simulink model "DKSTDD_DK_TuanTu_SG_Q_P_Y"  (R2019a)
settings: Solver=VariableStepAuto  StartTime=0.0  StopTime=10  RelTol=1e-3
libraries: powerlib x8
settings Model: Creator=Admin  LastModifiedBy=Admin
settings SolverCC: ZeroCrossAlgorithm=Adaptive
settings DebuggingCC: IgnoredZcDiagnostic=none

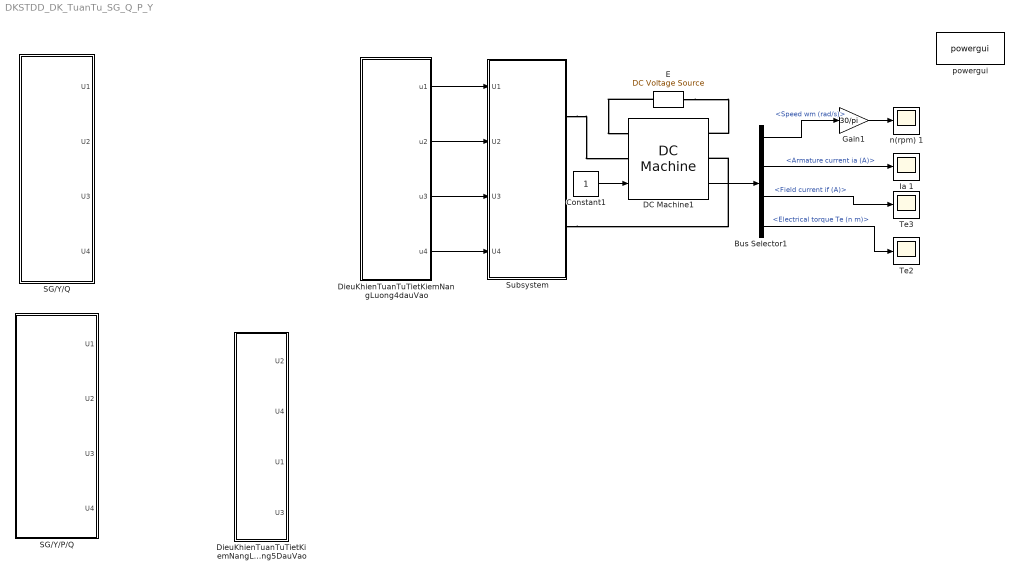
== system DKSTDD_DK_TuanTu_SG_Q_P_Y ==
  Bus Selector1 : BusSelector  OutputSignals=Speed wm (rad/s),Armature current ia (A),Field current if (A),Electrical torque Te (n m)
  Constant1 : Constant
  DC Machine1 : powerlib/Machines/DC Machine  PresetModel=01: 5HP 240V 1750RPM Field:300V  MechanicalLoad=Torque TL  FieldType=Wound  ShowDetailedParameters=on  MeasurementBus=off  RLa=[2.581 0.028]  RLf=[281.3 156]  Laf=0.9483  MachineConstant=Torque constant (N.m/A)  Ke=1.8  Kt=1.8  J=0.02215  Bm=0.002953  Tf=0.5161  w0=1  Ifinit=1  TsPowergui=0  TsBlock=-1
  "DieuKhienTuanTuTietKiemNangLuong4dauVao " : Subsystem
  "DieuKhienTuanTuTietKiemNangLuong5DauVao " : Subsystem
  E : powerlib/Electrical Sources/DC Voltage Source  Amplitude=300  Measurements=None
  Gain1 : Gain  Gain=30/pi
  Ia 1 : Scope
  SG/Y/P/Q : Subsystem
  SG/Y/Q : Subsystem
  Subsystem : Subsystem
  Te2 : Scope
  Te3 : Scope
  n(rpm) 1 : Scope
  powergui : powerlib/powergui  Priority=1  SimulationMode=Continuous  SampleTime=50e-6  frequency=60  Iterations=50  frequencyindice=0  Pbase=100e6  ErrMax=1e-4  UnitsV=kV  UnitsW=MW  buscounter=0  FunctionMessages=off  echomessages=off  EnableUseOfTLC=off  CurrentSourceSwitches=off  DisableSnubberDevices=off  DisableRonSwitches=off  DisableVfSwitches=off  DisplayEquations=off  AutomaticDiscreteSolvers=off  SolverType=Tustin/Backward Euler (TBE)  Interpol=off  ExternalGateDelay=off  methode=off  Ts=100  x0status=blocks  SPID=on  SwTol=0  HookPort=off  NonlinearTolerance=0  nMaxIteration=15  ContinueOnMaxIteration=off  RestoreLinks=warning  ResistiveCurrentMeasurement=off  Frange=[0:2:500]  Ylog=off  Xlog=on  ShowGrid=off  save=off  variable=ZData  structure=0  ZoomFFT=off  StartTime=0.0  cycles=1  DisplayStyle=1  fundamental=60  FreqAxis=off  MaxFrequency=1000  frequencyindicesteady=1  RmsSteady=1  display=off
      settings: SourceProductName=Simscape Electrical
  wires:
  Bus Selector1/4 -> Te2/1  "<Electrical torque Te (n m)>"
  Gain1/1 -> n(rpm) 1/1
  DC Machine1/1 -> Bus Selector1/1
  Bus Selector1/3 -> Te3/1  "<Field current if (A)>"
  Bus Selector1/1 -> Gain1/1  "<Speed wm (rad/s)>"
  Constant1/1 -> DC Machine1/1
  Bus Selector1/2 -> Ia 1/1  "<Armature current ia (A)>"
  "DieuKhienTuanTuTietKiemNangLuong4dauVao "/1(u1) -> Subsystem/1(U1)
  "DieuKhienTuanTuTietKiemNangLuong4dauVao "/2("u2 ") -> Subsystem/2(U2)
  "DieuKhienTuanTuTietKiemNangLuong4dauVao "/3(u3) -> Subsystem/3(U3)
  "DieuKhienTuanTuTietKiemNangLuong4dauVao "/4(u4) -> Subsystem/4(U4)
  connections:
  E/RConn1 -- DC Machine1/LConn2
  Subsystem/RConn2 -- DC Machine1/RConn1
  Subsystem/RConn1 -- DC Machine1/LConn1
  E/LConn1 -- DC Machine1/RConn2

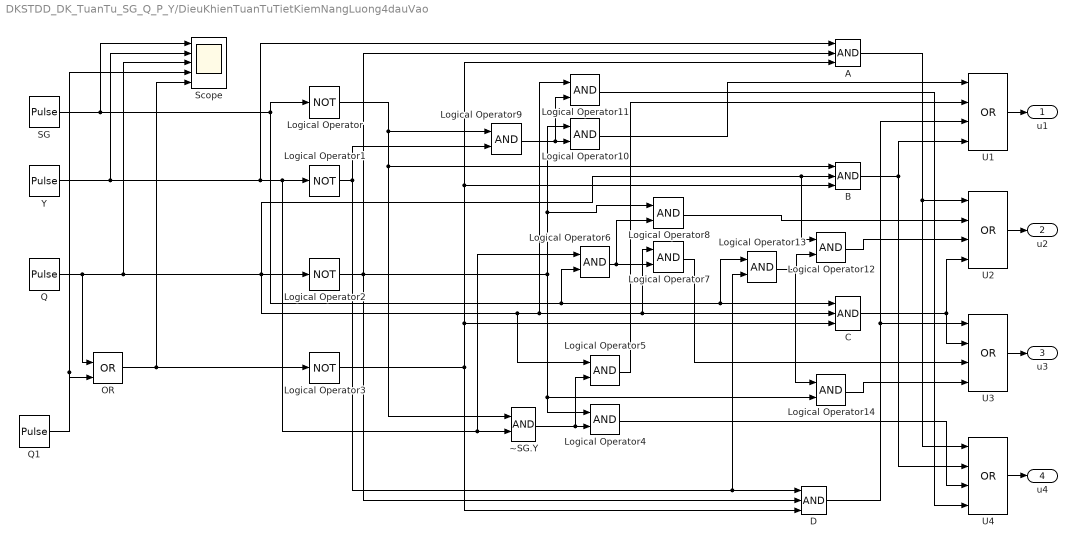
== system DKSTDD_DK_TuanTu_SG_Q_P_Y/DieuKhienTuanTuTietKiemNangLuong4dauVao  ==
  A : Logic  Inputs=3  AllPortsSameDT=off  OutDataTypeStr=boolean
  B : Logic  Inputs=3  AllPortsSameDT=off  OutDataTypeStr=boolean
  C : Logic  Inputs=3  AllPortsSameDT=off  OutDataTypeStr=boolean
  D : Logic  Inputs=3  AllPortsSameDT=off  OutDataTypeStr=boolean
  Logical Operator{,1..3} (4 alike) : Logic  Operator=NOT  AllPortsSameDT=off  OutDataTypeStr=boolean
  Logical Operator{4..14} (11 alike) : Logic  AllPortsSameDT=off  OutDataTypeStr=boolean
  OR : Logic  Operator=OR  IconShape=distinctive  AllPortsSameDT=off  OutDataTypeStr=boolean
  Q : DiscretePulseGenerator  PulseType=Time based  Period=0.002  PulseWidth=70
  Q1 : DiscretePulseGenerator  PulseType=Time based  Period=0.002  PulseWidth=70  PhaseDelay=0.0022
  SG : DiscretePulseGenerator  PulseType=Time based  Period=0.008  PulseWidth=50  PhaseDelay=0.008
  Scope : Scope  NumInputPorts=5
  U{1..4} (4 alike) : Logic  Operator=OR  Inputs=4  AllPortsSameDT=off  OutDataTypeStr=boolean
  Y : DiscretePulseGenerator  PulseType=Time based  Period=0.004  PulseWidth=50  PhaseDelay=0.002
  ~SG.Y : Logic  AllPortsSameDT=off  OutDataTypeStr=boolean
  u1 : Outport
  "u2 " : Outport  Port=2
  u3 : Outport  Port=3
  u4 : Outport  Port=4
  wires:
  Logical Operator3/1 -> D/3, C/3, B/3, A/3
  Logical Operator6/1 -> Logical Operator7/2, Logical Operator8/2
  Logical Operator9/1 -> Logical Operator11/2, Logical Operator10/2
  Q/1 -> OR/1, Scope/3, C/2, Logical Operator7/1, Logical Operator11/1, Logical Operator5/1, Logical Operator12/1, B/2, Logical Operator2/1
  B/1 -> U4/2, U1/4
  Logical Operator8/1 -> U2/2
  Logical Operator10/1 -> U1/1
  Logical Operator/1 -> ~SG.Y/1, B/1, Logical Operator9/1
  A/1 -> U4/1, U2/1
  Logical Operator7/1 -> U3/3
  SG/1 -> Scope/1, Logical Operator/1, C/1, Logical Operator13/1, Logical Operator6/2
  Logical Operator2/1 -> Logical Operator4/1, Logical Operator14/2, Logical Operator10/1, Logical Operator8/1, D/2, A/2
  ~SG.Y/1 -> Logical Operator5/2, Logical Operator4/2
  OR/1 -> Scope/5, Logical Operator3/1
  U4/1 -> u4/1
  Y/1 -> Scope/2, A/1, ~SG.Y/2, Logical Operator6/1, Logical Operator1/1
  Logical Operator5/1 -> U1/2
  D/1 -> U3/1, U1/3
  U3/1 -> u3/1
  Logical Operator1/1 -> Logical Operator9/2, Logical Operator13/2, D/1
  Logical Operator4/1 -> U4/3
  C/1 -> U3/2, U2/4
  Logical Operator14/1 -> U3/4
  Logical Operator11/1 -> U4/4
  Logical Operator13/1 -> Logical Operator14/1, Logical Operator12/2
  Logical Operator12/1 -> U2/3
  U2/1 -> "u2 "/1
  U1/1 -> u1/1
  Q1/1 -> OR/2, Scope/4

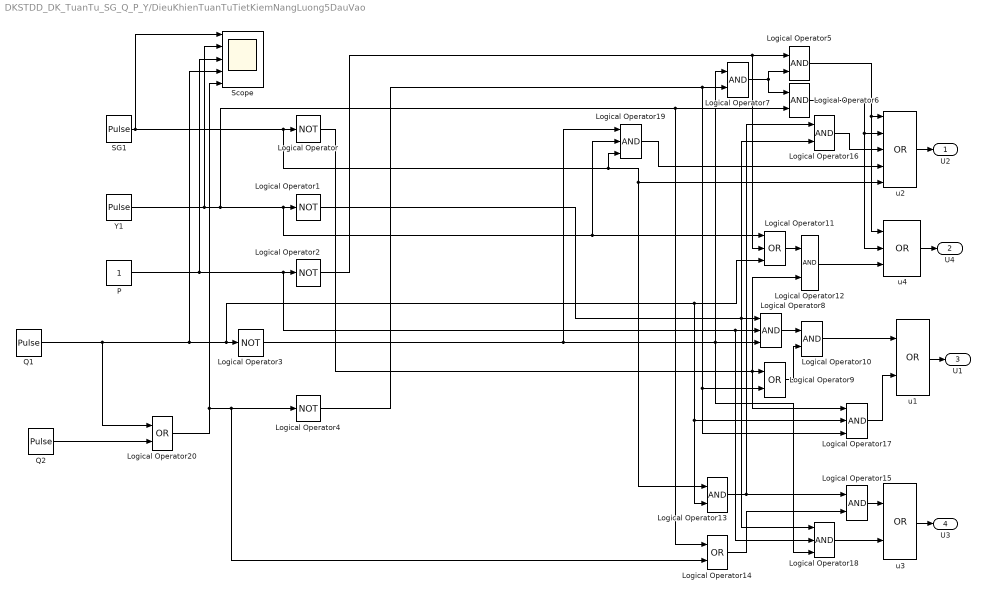
== system DKSTDD_DK_TuanTu_SG_Q_P_Y/DieuKhienTuanTuTietKiemNangLuong5DauVao  ==
  Logical Operator{,1..4} (5 alike) : Logic  Operator=NOT  AllPortsSameDT=off  OutDataTypeStr=boolean
  Logical Operator{5..7,10,12..13,15..16} (8 alike) : Logic  AllPortsSameDT=off  OutDataTypeStr=boolean
  Logical Operator11 : Logic  Operator=OR  Inputs=3  AllPortsSameDT=off  OutDataTypeStr=boolean
  Logical Operator14 : Logic  Operator=OR  AllPortsSameDT=off  OutDataTypeStr=boolean
  Logical Operator{8,17..19} (4 alike) : Logic  Inputs=3  AllPortsSameDT=off  OutDataTypeStr=boolean
  Logical Operator20 : Logic  Operator=OR  AllPortsSameDT=off  OutDataTypeStr=boolean
  Logical Operator9 : Logic  Operator=OR  AllPortsSameDT=off  OutDataTypeStr=boolean
  P : Constant
  Q1 : DiscretePulseGenerator  PulseType=Time based  Period=0.002  PulseWidth=70
  Q2 : DiscretePulseGenerator  PulseType=Time based  Period=0.002  PulseWidth=70  PhaseDelay=0.0021
  SG1 : DiscretePulseGenerator  PulseType=Time based  Period=0.008  PulseWidth=50  PhaseDelay=0.008
  Scope : Scope  NumInputPorts=5
  Y1 : DiscretePulseGenerator  PulseType=Time based  Period=0.004  PulseWidth=50  PhaseDelay=0.002
  u1 : Logic  Operator=OR  AllPortsSameDT=off  OutDataTypeStr=boolean
  u2 : Logic  Operator=OR  Inputs=5  AllPortsSameDT=off  OutDataTypeStr=boolean
  u3 : Logic  Operator=OR  AllPortsSameDT=off  OutDataTypeStr=boolean
  u4 : Logic  Operator=OR  Inputs=3  AllPortsSameDT=off  OutDataTypeStr=boolean
  U2 : Outport
  U4 : Outport  Port=2
  U1 : Outport  Port=3
  U3 : Outport  Port=4
  wires:
  u4/1 -> U4/1
  SG1/1 -> Scope/1, Logical Operator19/3, u2/5, Logical Operator13/1, Logical Operator/1
  Logical Operator/1 -> Logical Operator12/2, Logical Operator9/1, Logical Operator17/1
  Logical Operator5/1 -> u4/1, u2/1
  Logical Operator13/1 -> Logical Operator16/1, Logical Operator15/1
  Logical Operator18/1 -> u3/2
  Logical Operator20/1 -> Scope/5, Logical Operator14/2, Logical Operator4/1
  Logical Operator2/1 -> Logical Operator11/2, Logical Operator5/1
  Logical Operator1/1 -> Logical Operator8/1, Logical Operator16/2, Logical Operator18/1
  Logical Operator10/1 -> u1/1
  Logical Operator15/1 -> u3/1
  P/1 -> Logical Operator18/2, Logical Operator8/2, Logical Operator2/1, Scope/3
  Q1/1 -> Logical Operator20/1, Logical Operator13/2, Logical Operator17/2, Logical Operator11/3, Logical Operator3/1, Scope/4
  Logical Operator14/1 -> Logical Operator15/2
  Logical Operator6/1 -> u4/2, u2/2
  Logical Operator3/1 -> Logical Operator8/3, Logical Operator7/1, Logical Operator18/3, Logical Operator19/1
  Y1/1 -> Logical Operator6/2, Logical Operator14/1, Logical Operator11/1, Logical Operator19/2, Logical Operator1/1, Scope/2
  Logical Operator4/1 -> Logical Operator9/2, Logical Operator17/3, Logical Operator7/2
  Logical Operator16/1 -> u2/3
  Logical Operator7/1 -> Logical Operator5/2, Logical Operator6/1
  Logical Operator11/1 -> Logical Operator12/1
  Logical Operator8/1 -> Logical Operator10/1
  Logical Operator9/1 -> Logical Operator10/2
  Logical Operator19/1 -> u2/4
  Logical Operator17/1 -> u1/2
  Logical Operator12/1 -> u4/3
  u1/1 -> U1/1
  u2/1 -> U2/1
  u3/1 -> U3/1
  Q2/1 -> Logical Operator20/2

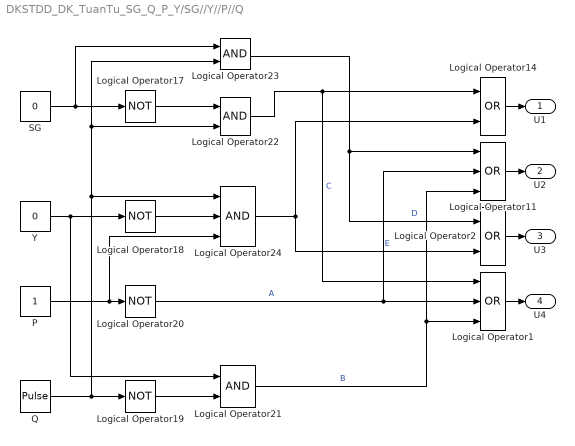
== system DKSTDD_DK_TuanTu_SG_Q_P_Y/SG//Y//P//Q ==
  Logical Operator1 : Logic  Operator=OR  Inputs=3  AllPortsSameDT=off  OutDataTypeStr=boolean
  Logical Operator11 : Logic  Operator=OR  Inputs=3  AllPortsSameDT=off  OutDataTypeStr=boolean
  Logical Operator14 : Logic  Operator=OR  AllPortsSameDT=off  OutDataTypeStr=boolean
  Logical Operator{17..20} (4 alike) : Logic  Operator=NOT  AllPortsSameDT=off  OutDataTypeStr=boolean
  Logical Operator2 : Logic  Operator=OR  AllPortsSameDT=off  OutDataTypeStr=boolean
  Logical Operator21 : Logic  AllPortsSameDT=off  OutDataTypeStr=boolean
  Logical Operator22 : Logic  AllPortsSameDT=off  OutDataTypeStr=boolean
  Logical Operator23 : Logic  AllPortsSameDT=off  OutDataTypeStr=boolean
  Logical Operator24 : Logic  Inputs=3  AllPortsSameDT=off  OutDataTypeStr=boolean
  P : Constant
  Q : DiscretePulseGenerator  PulseType=Time based  Period=0.002  PulseWidth=80
  SG : Constant  Value=0
  Y : Constant  Value=0
  U1 : Outport
  U2 : Outport  Port=2
  U3 : Outport  Port=3
  U4 : Outport  Port=4
  wires:
  P/1 -> Logical Operator24/3, Logical Operator20/1
  Logical Operator19/1 -> Logical Operator21/2
  Logical Operator1/1 -> U4/1
  Q/1 -> Logical Operator23/2, Logical Operator22/2, Logical Operator24/1, Logical Operator19/1
  Logical Operator18/1 -> Logical Operator24/2
  Y/1 -> Logical Operator21/1, Logical Operator18/1
  SG/1 -> Logical Operator23/1, Logical Operator17/1
  Logical Operator20/1 -> Logical Operator1/2, Logical Operator11/2  "A"
  Logical Operator23/1 -> Logical Operator2/1, Logical Operator11/1  "D"
  Logical Operator17/1 -> Logical Operator22/1
  Logical Operator22/1 -> Logical Operator1/1, Logical Operator14/1  "C"
  Logical Operator21/1 -> Logical Operator1/3, Logical Operator11/3  "B"
  Logical Operator24/1 -> Logical Operator2/2, Logical Operator14/2  "E"
  Logical Operator11/1 -> U2/1
  Logical Operator14/1 -> U1/1
  Logical Operator2/1 -> U3/1

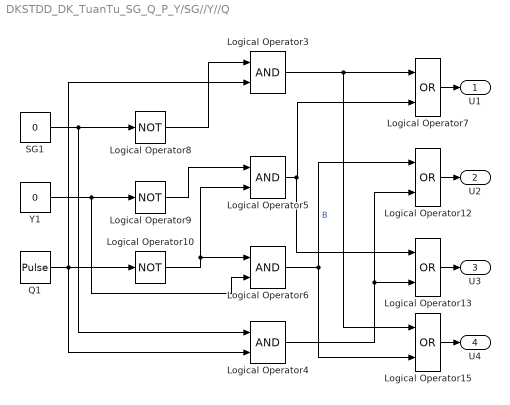
== system DKSTDD_DK_TuanTu_SG_Q_P_Y/SG//Y//Q ==
  Logical Operator10 : Logic  Operator=NOT  AllPortsSameDT=off  OutDataTypeStr=boolean
  Logical Operator{7,12..13,15} (4 alike) : Logic  Operator=OR  AllPortsSameDT=off  OutDataTypeStr=boolean
  Logical Operator{3..6} (4 alike) : Logic  AllPortsSameDT=off  OutDataTypeStr=boolean
  Logical Operator8 : Logic  Operator=NOT  AllPortsSameDT=off  OutDataTypeStr=boolean
  Logical Operator9 : Logic  Operator=NOT  AllPortsSameDT=off  OutDataTypeStr=boolean
  Q1 : DiscretePulseGenerator  PulseType=Time based  Period=0.002  PulseWidth=60
  SG1 : Constant  Value=0
  Y1 : Constant  Value=0
  U1 : Outport
  U2 : Outport  Port=2
  U3 : Outport  Port=3
  U4 : Outport  Port=4
  wires:
  Q1/1 -> Logical Operator4/2, Logical Operator3/2, Logical Operator10/1
  SG1/1 -> Logical Operator4/1, Logical Operator8/1
  Logical Operator12/1 -> U2/1
  Logical Operator5/1 -> Logical Operator13/1, Logical Operator7/2
  Logical Operator8/1 -> Logical Operator3/1
  Logical Operator4/1 -> Logical Operator13/2, Logical Operator12/2
  Logical Operator3/1 -> Logical Operator15/1, Logical Operator7/1
  Y1/1 -> Logical Operator6/2, Logical Operator9/1
  Logical Operator10/1 -> Logical Operator6/1, Logical Operator5/2
  Logical Operator6/1 -> Logical Operator15/2, Logical Operator12/1  "B"
  Logical Operator9/1 -> Logical Operator5/1
  Logical Operator15/1 -> U4/1
  Logical Operator7/1 -> U1/1
  Logical Operator13/1 -> U3/1

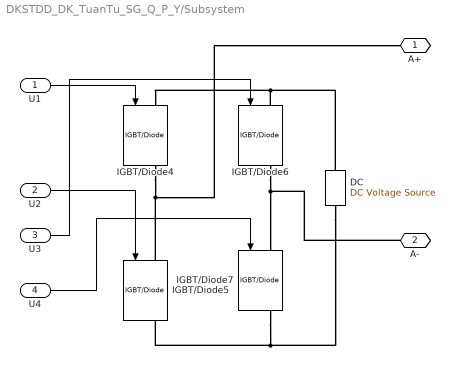
== system DKSTDD_DK_TuanTu_SG_Q_P_Y/Subsystem ==
  U1 : Inport
  U2 : Inport  Port=2
  U3 : Inport  Port=3
  U4 : Inport  Port=4
  DC : powerlib/Electrical Sources/DC Voltage Source  Amplitude=240  Measurements=None
  IGBT/Diode{4..7} (4 alike) : powerlib/Power Electronics/IGBT//Diode  Ron=1e-3  Rs=1e5  Cs=inf  Measurements=on
      settings: SourceProductName=Simscape Electrical
  A+ : PMIOPort  Side=Right
  A- : PMIOPort  Port=2  Side=Right
  wires:
  U1/1 -> IGBT/Diode4/1
  U4/1 -> IGBT/Diode7/1
  U2/1 -> IGBT/Diode5/1
  U3/1 -> IGBT/Diode6/1
  connections:
  IGBT/Diode5/LConn1 -- IGBT/Diode4/RConn1 -- A+/RConn1
  DC/RConn1 -- IGBT/Diode6/LConn1 -- IGBT/Diode4/LConn1
  IGBT/Diode6/RConn1 -- A-/RConn1 -- IGBT/Diode7/LConn1
  DC/LConn1 -- IGBT/Diode7/RConn1 -- IGBT/Diode5/RConn1
